simulink model "FOC_CHBI"  (R2025a)
settings: Solver=VariableStepAuto  StartTime=0.0  StopTime=6.5  RelTol=1e-3
InitFcn:
  | %% KHOI THONG SO DONG CO
  | U_nom=6000;%6600;           %dien ap dinh muc dong co
  | H=0.96;%0.9387;             %hieu suat dong co
  | Pn=1e6;%1750e3;         %Cong suat dinh muc dong co
  | cosphi=0.85;%0.9297;        %He so cong suat
  | Sn=Pn/cosphi;       %Cong suat toan phan
  | J=27.9;%34.8;                %Moment quan tinh
  | pc=2;%2;               %So cap cuc
  | fn=50;              %Tan so luoi
  | n=1490;%1486;             %Toc do dinh muc 2880
  | Mdm=6153;%(9.55*Pn*H)/n;  %Moment dinh muc
  | In=117;%Pn/(U_nom*H*cosphi*sqrt(3))   ;
  | Isd=sqrt(2)*In*sqrt(1-cosphi);
  | Isq=sqrt(2*In^2-Isd^2);
  | wrn=2*pi*(fn-(pc*n/60));               %Toc do truotdinh muc
  | Tr=Isq/(wrn*Isd) ;                   %Tinh 'Tr'trong cac cong thuc
  | %Xo=(sqrt(1-cosphi^2)-cosphi*Isd/Isq)*(Un*sqrt(2)/(sqrt(3)*In));
  | Xo=(sqrt(1-cosphi^2)-cosphi*Isd/Isq)*(U_nom/(sqrt(3)*In));
  | Xh=sqrt(2/3)*(U_nom/Isd) - Xo;
  | Rs=(wrn*Isd*Xh)/(2*pi*fn*Isq);
  | Rr=Rs;
  | o=Xo/Xh;
  | Ts=Xh/(2*pi*fn*Rs);
  | Tos=o*Ts;
  | Lr=Tr*Rr;
  | Lor=o*Lr;
  | Ls=Ts*Rs;
  | Los=o*Ls;
  | Lm=sqrt((1-o)*Ls*Lr);
  | %tham so dong co 2850e3Kw
  | %Rs=0.05;
  | %Rr = 0.062;
  | %Los = 0.957/(100*pi);
  | %Lor = 2.237/(100*pi);
  | %Lm = 34.826/(100*pi);
  | %Ts = (Lm +Los)/Rs;
  | %Tr = (Lm+Lor)/Rr;
  | %Lr = Lm + Lor;
  | %Ls = Lm + Los;
  | Udc = 1.1*6000/(0.612*12);%6600/(0.612*12);
  | Rt =18*Udc*Udc/1e6; %18*Udc*Udc/2010.6e3;
  | C_f = 5/(6*100*pi*Rt*0.001);
  | %Fan and Pumb Load Coeficient
  | TL0 = (2.0/100)*Mdm; %(2.0/100)*TN;
  | Omega_rated = n/9.55; %nN/9.55; %rad/s
  | LoadGain = (Mdm - TL0)/(Omega_rated*Omega_rated);
  | fs=5000;
  | %% THAM SO CAC BO DIEU KHIEN
  | %---------------- control volocity
  | epxilon = 0.7;
  | wn = 40;
  |      %P_w = (2*epxilon*wn*J)/pc;
  |     %I_w = wn*wn*J/pc;
  |  P_w = 60;%5;%15;%9;%12;%10;%(2*epxilon*wn*J)/pc
  |  I_w = 80;%150;%80;%100;%40;%50;%wn*wn*J/pc
  | %---------------- control current
  |     %P_id = Rs*Tos*fs/5;
  |     % I_id = Rs*Tos*fs/5/Tos;
  |      %P_iq = P_id;
  |      %I_iq = I_id;
  | P_id = 50;%50;%25;%25;%Rs*Tos*1500/5
  |  I_id = 5000;%5000;%9860;%Rs*Tos*1500/5/Tos
  |  P_iq = 50;%50;%P_id;
  |  I_iq = 5000;%I_id;
  | % --------------control torque
  |  I_phi = 10;%37;%Tr/(5*Tos)/Tr
  |  P_phi = 200;%5;%Tr/(5*Tos)
  |      %I_phi = Tr/(5);
  |      %P_phi = Tr*fs/(5);
StopFcn:
  | figure(1);
  | subplot(1,1,1); hold on; grid on;
  | plot(phi_ref.time, phi_ref.signals.values,'r--', 'Linewidth',1.5);
  | plot(phi.time, phi.signals.values,'b', 'Linewidth',1.5);
  | legend('phi*-rd','phi-rd');
  | title('Từ thông');
  | xlabel('Thời gian (s)'); ylabel('Wb');
  | 
  | 
  | figure(2);
  | subplot(2,1,1); hold on; grid on;
  | plot(torque.time, torque.signals.values,'r','Linewidth',1.5);
  | legend('Te');
  | title('Mô-men');
  | xlabel('Thời gian (s)'); ylabel('Nm');
  | 
  | subplot(2,1,2); hold on; grid on;
  | plot(speed_ref.time, speed_ref.signals.values,'r--','Linewidth',1.5);
  | plot(speed.time, speed.signals.values,'b','Linewidth',1.5);
  | legend('Tốc độ đặt','Tốc độ thực');
  | title('Tốc độ');
  | xlabel('Thời gian (s)'); ylabel('RPM');
  | 
  | figure(3)
  | 
  | subplot(2,1,1); hold on; grid on;
  | plot(isd_ref.time, isd_ref.signals.values,'r','Linewidth',1.5);
  | plot(isd.time, isd.signals.values,'b','Linewidth',1.5);
  | legend('isd*','isd');
  | title('Dòng điện isd');
  | xlabel('Thời gian (s)'); ylabel('A');
  | 
  | subplot(2,1,2); hold on; grid on;
  | plot(isq_ref.time, isq_ref.signals.values,'r','Linewidth',1.5);
  | plot(isq.time, isq.signals.values,'b','Linewidth',1.5);
  | legend('isq*','isq');
  | title('Dòng điện isq');
  | xlabel('Thời gian (s)'); ylabel('A');
  | 
  | figure(4)
  | 
  | subplot(2,1,1); hold on; grid on;
  | plot(va.time, va.signals.values,'b','Linewidth',1.5);
  | plot(vb.time, vb.signals.values,'k','Linewidth',1.5);
  | plot(vc.time, vc.signals.values,'r','Linewidth',1.5);
  | legend('Ua','Ub','Uc');
  | title('Điện áp pha');
  | xlabel('Thời gian (s)'); ylabel('V');
  | 
  | subplot(2,1,2); hold on; grid on;
  | plot(vab.time, vab.signals.values,'k','Linewidth',1.5);
  | plot(vbc.time, vbc.signals.values,'b','Linewidth',1.5);
  | plot(vca.time, vca.signals.values,'r','Linewidth',1.5);
  | legend('Uab','Ubc','Uca');
  | title('Điện áp dây');
  | xlabel('Thời gian (s)'); ylabel('V');
  | 
  | figure(5);
  | subplot(1,1,1); hold on; grid on;
  | plot(Ia.time, Ia.signals.values,'k','Linewidth',1.5);
  | plot(Ib.time, Ib.signals.values,'b','Linewidth',1.5);
  | plot(Ic.time, Ic.signals.values,'r','Linewidth',1.5);
  | legend('Ia','Ib','Ic');
  | title('Dòng điện ba pha của động cơ');
  | xlabel('Thời gian (s)'); ylabel('A');
undefined symbols (not defined in the file): sigbuilder_block
libraries: spsIGBTDiodeLib x72, spsTriangleGeneratorLib x36, spsSeriesRLCBranchLib x18, spsBreakerLib x18, spsUniversalBridgeLib x18, spsZigzagPhaseShiftingTransformerLib x15, spsVoltageMeasurementLib x8, spsACVoltageSourceLib x3, spsCurrentMeasurementLib x3, spsThreePhaseTransformerTwoWindingsLib x3, slpidlib x2, spsThreePhaseVIMeasurementLib x1
(part 1 of 3)
settings Model: Creator=Admin  LastModifiedBy=HP
settings SolverCC: AlgebraicLoopSolver=TrustRegion
settings DataIOCC: ReturnWorkspaceOutputs=off
settings OptimizationCC: ReuseModelBlockBuffer=off
settings DebuggingCC: ArithmeticOperatorsInVariantConditions=warning
settings SFSimCC: CustomCodeUndefinedFunction=UseInterfaceOnly
settings RTWCC: GPUComputeCapability=3.5

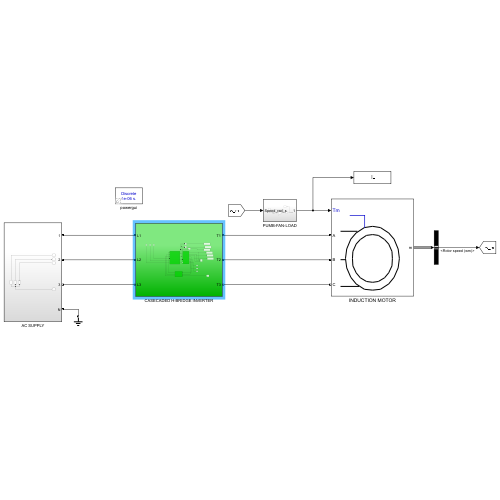
[thumbnail: Simulink's stored preview of the top-level diagram]
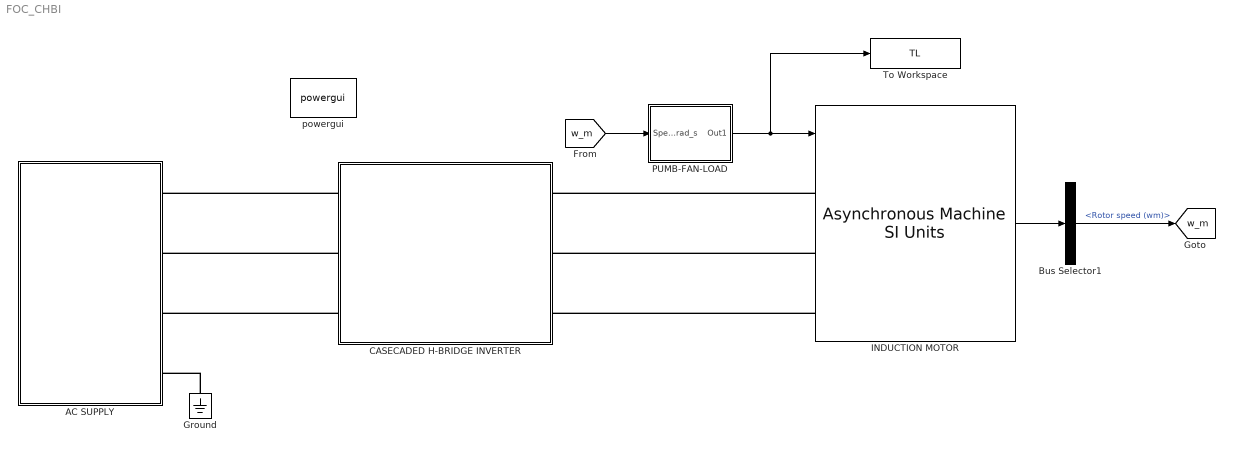
== system FOC_CHBI ==
  AC SUPPLY : Subsystem
  Bus Selector1 : BusSelector  OutputSignals=Mechanical.Rotor speed (wm)
  CASECADED H-BRIDGE INVERTER : Subsystem
  Ground : spsGroundLib/Ground  LConnTagsString=a
  INDUCTION MOTOR : spsAsynchronousMachineSIUnitsLib/Asynchronous Machine SI Units  RotorType=Squirrel-cage  PresetModel=No  MechanicalLoad=Torque Tm  ShowDetailedParameters=on  ReferenceFrame=Rotor  Units=SI  MeasurementBus=off  NominalParameters=[Pn U_nom fn]  VoltageRatio=1  Stator=[Rs Los]  Rotor=[Rr Lor]  Cage1=[ 0.022 0.226/377]  Cage2=[ 0.022 0.226/377]  Lm=Lm  Mechanical=[J 0 pc]  PolePairs=2  InitialConditions=[1,0,0,0,0,0,0,0]  SimulateSaturation=off  Saturation=[0 0;0 0]  LoadFlowParameters=0  TsPowergui=0  TsBlock=-1  IterativeModel=Forward Euler  IterativeDiscreteModel=Trapezoidal non iterative  Pmec=0
      settings: AttributesFormatString=\n
  PUMB-FAN-LOAD : Subsystem
  To Workspace : ToWorkspace  VariableName=TL  SaveFormat=Structure With Time  SampleTime=-1
  powergui : sps_lib/powergui  Priority=1  SimulationMode=Discrete  SampleTime=1e-6  frequency=60  Iterations=50  frequencyindice=0  Pbase=100e6  ErrMax=1e-4  UnitsV=kV  UnitsW=MW  buscounter=0  FunctionMessages=off  echomessages=off  EnableUseOfTLC=off  CurrentSourceSwitches=off  DisableSnubberDevices=off  DisableRonSwitches=off  DisableVfSwitches=off  DisplayEquations=off  AutomaticDiscreteSolvers=off  SolverType=Tustin  Interpol=off  ExternalGateDelay=off  methode=off  Ts=0  x0status=blocks  SPID=on  SwTol=0  HookPort=off  NonlinearTolerance=1e-4  nMaxIteration=100  ContinueOnMaxIteration=off  RestoreLinks=warning  ResistiveCurrentMeasurement=off  Frange=[0:2:500]  Ylog=off  Xlog=on  ShowGrid=off  save=off  variable=ZData  structure=Is  ZoomFFT=off  StartTime=0.8  cycles=5  DisplayStyle=1  fundamental=50  FreqAxis=off  MaxFrequency=1000  frequencyindicesteady=1  RmsSteady=1  display=off
  tag scope: w_m=global
  wires:
  [w_m] -> PUMB-FAN-LOAD/1(Speed_rad_s)
  PUMB-FAN-LOAD/1(Out1) -> To Workspace/1, INDUCTION MOTOR/1
  Bus Selector1/1 -> [w_m]  "<Rotor speed (wm)>"
  INDUCTION MOTOR/1 -> Bus Selector1/1
  connections:
  CASECADED H-BRIDGE INVERTER/LConn3 -- AC SUPPLY/RConn3
  CASECADED H-BRIDGE INVERTER/LConn1 -- AC SUPPLY/RConn1
  INDUCTION MOTOR/LConn2 -- CASECADED H-BRIDGE INVERTER/RConn2
  INDUCTION MOTOR/LConn3 -- CASECADED H-BRIDGE INVERTER/RConn3
  INDUCTION MOTOR/LConn1 -- CASECADED H-BRIDGE INVERTER/RConn1
  Ground/LConn1 -- AC SUPPLY/RConn4
  CASECADED H-BRIDGE INVERTER/LConn2 -- AC SUPPLY/RConn2

== system FOC_CHBI/AC SUPPLY ==
  Va : spsACVoltageSourceLib/AC Voltage Source  Description=source block  Amplitude=sqrt(2)*U_nom/sqrt(3)  Phase=0  Frequency=50  SampleTime=1e-5  Measurements=None  BusType=swing  Pref=10e3  Qref=0  Qmin=-inf  Qmax=+inf
      settings: AttributesFormatString=\n
  Vb : spsACVoltageSourceLib/AC Voltage Source  Description=source block  Amplitude=sqrt(2)*U_nom/sqrt(3)  Phase=-120  Frequency=50  SampleTime=1e-5  Measurements=None  BusType=swing  Pref=10e3  Qref=0  Qmin=-inf  Qmax=+inf
      settings: AttributesFormatString=\n
  Vc : spsACVoltageSourceLib/AC Voltage Source  Description=source block  Amplitude=sqrt(2)*U_nom/sqrt(3)  Phase=120  Frequency=50  SampleTime=1e-5  Measurements=None  BusType=swing  Pref=10e3  Qref=0  Qmin=-inf  Qmax=+inf
      settings: AttributesFormatString=\n
  Connection Port : PMIOPort  Tag=PMCPort  Side=Right
  Connection Port1 : PMIOPort  Tag=PMCPort  Port=2  Side=Right
  Connection Port2 : PMIOPort  Tag=PMCPort  Port=3  Side=Right
  N : PMIOPort  Tag=PMCPort  Port=4  Side=Right
  connections:
  Va/RConn1 -- Connection Port/RConn1
  Vb/RConn1 -- Connection Port1/RConn1
  Vc/RConn1 -- Connection Port2/RConn1
  Va/LConn1 -- N/RConn1 -- Vc/LConn1 -- Vb/LConn1

== system FOC_CHBI/CASECADED H-BRIDGE INVERTER ==
  CONTROLLER : Subsystem
  MEASUREMENT : Subsystem
  POWER CIRCUIT1 : Subsystem
  Scope : Scope  NumInputPorts=3
      settings: Title=Điện áp pha  ActiveDisplayYMinimum=-4924.2153222862125  ActiveDisplayYMaximum=5141.53101611316  YLabel=V
  To Workspace : ToWorkspace  VariableName=vab  SaveFormat=Structure With Time  SampleTime=-1
  To Workspace1 : ToWorkspace  VariableName=va  SaveFormat=Structure With Time  SampleTime=-1
  To Workspace2 : ToWorkspace  VariableName=vbc  SaveFormat=Structure With Time  SampleTime=-1
  To Workspace3 : ToWorkspace  VariableName=vca  SaveFormat=Structure With Time  SampleTime=-1
  To Workspace4 : ToWorkspace  VariableName=vb  SaveFormat=Structure With Time  SampleTime=-1
  To Workspace5 : ToWorkspace  VariableName=vc  SaveFormat=Structure With Time  SampleTime=-1
  Vab : spsVoltageMeasurementLib/Voltage Measurement  PhasorSimulation=off  OutputType=Complex  PSBequivalent=0
  Vbc : spsVoltageMeasurementLib/Voltage Measurement  PhasorSimulation=off  OutputType=Complex  PSBequivalent=0
  Vca : spsVoltageMeasurementLib/Voltage Measurement  PhasorSimulation=off  OutputType=Complex  PSBequivalent=0
  L1 : PMIOPort  Side=Left
  L2 : PMIOPort  Port=2  Side=Left
  L3 : PMIOPort  Port=3  Side=Left
  T1 : PMIOPort  Port=4  Side=Right
  T2 : PMIOPort  Port=5  Side=Right
  T3 : PMIOPort  Port=6  Side=Right
  wires:
  MEASUREMENT/5(iB) -> CONTROLLER/2(Ib)
  [w_m] -> CONTROLLER/3(w)
  MEASUREMENT/4(iA) -> CONTROLLER/1(Ia)
  CONTROLLER/1(phaa) -> POWER CIRCUIT1/1(phaa)
  CONTROLLER/2(phab) -> POWER CIRCUIT1/2(phab)
  CONTROLLER/3(phac) -> POWER CIRCUIT1/3(phac)
  MEASUREMENT/1(Van) -> To Workspace1/1, Scope/1
  MEASUREMENT/2(Vbn) -> Scope/2, To Workspace4/1
  MEASUREMENT/3(Vcn) -> To Workspace5/1, Scope/3
  Vab/1 -> To Workspace/1
  Vbc/1 -> To Workspace2/1
  Vca/1 -> To Workspace3/1
  connections:
  POWER CIRCUIT1/LConn1 -- L1/RConn1
  POWER CIRCUIT1/LConn2 -- L2/RConn1
  POWER CIRCUIT1/LConn3 -- L3/RConn1
  T2/RConn1 -- MEASUREMENT/RConn2
  T3/RConn1 -- MEASUREMENT/RConn3
  T1/RConn1 -- MEASUREMENT/RConn1
  POWER CIRCUIT1/RConn1 -- Vab/LConn1 -- Vca/LConn2 -- MEASUREMENT/LConn1
  POWER CIRCUIT1/RConn2 -- Vab/LConn2 -- Vbc/LConn1 -- MEASUREMENT/LConn2
  POWER CIRCUIT1/RConn3 -- Vbc/LConn2 -- Vca/LConn1 -- MEASUREMENT/LConn3
  POWER CIRCUIT1/RConn4 -- MEASUREMENT/LConn4

== system FOC_CHBI/PUMB-FAN-LOAD ==
  Speed_rad_s : Inport
  Add : Sum
  Constant1 : Constant  Value=TL0
  Gain : Gain  Gain=LoadGain
  Product : Product
  Out1 : Outport  VectorParamsAs1DForOutWhenUnconnected=off
  tag scope: TL=global
  wires:
  Constant1/1 -> Add/1
  Product/1 -> Gain/1
  Gain/1 -> Add/2
  Add/1 -> [TL], Out1/1
  Speed_rad_s/1 -> Product/1, Product/2

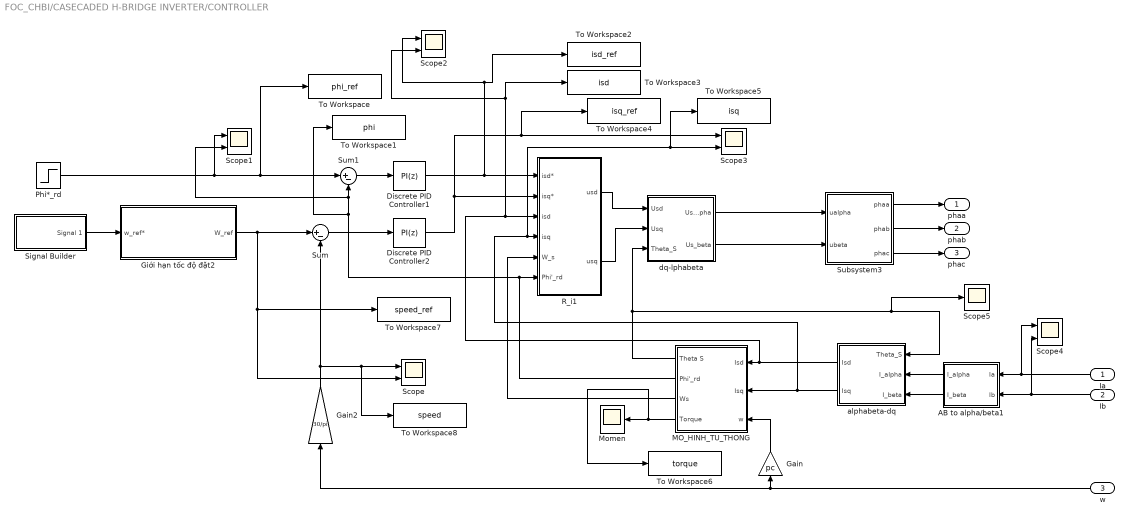
== system FOC_CHBI/CASECADED H-BRIDGE INVERTER/CONTROLLER ==
  Ia : Inport
  Ib : Inport  Port=2
  w : Inport  Port=3
  AB to alpha/beta1 : Subsystem
  Discrete PID Controller1 : slpidlib/PID Controller  Controller=PI  Form=Parallel  TimeDomain=Discrete-time  UseExternalTs=off  SampleTime=1/5e5  IntegratorMethod=Forward Euler  FilterMethod=Forward Euler  ControllerParametersSource=internal  P=P_phi  I=I_phi  UseKiTs=off  D=0  UseExternalDerivativeSource=off  N=100  UseFilter=on  TunerSelectOption=Transfer Function Based (PID Tuner App)  InitialConditionSource=internal  InitialConditionForIntegrator=0  InitialConditionForFilter=0  DifferentiatorICPrevScaledInput=0  ExternalReset=none  TrackingMode=off  Kt=1  LimitOutput=on  SatLimitsSource=internal  UpperSaturationLimit=1.8*Isd  LowerSaturationLimit=-1.8*Isd  LinearizeAsGain=off  AntiWindupMode=clamping  Kb=1  LimitIntegrator=off  UpperIntegratorSaturationLimit=inf  LowerIntegratorSaturationLimit=-inf  POutMin=[]  POutMax=[]  IOutMin=[]  IOutMax=[]  DOutMin=[]  DOutMax=[]  NOutMin=[]  NOutMax=[]  SumOutMin=[]  SumOutMax=[]  SaturationOutMin=[]  SaturationOutMax=[]  PParamMin=[]  PParamMax=[]  IParamMin=[]  IParamMax=[]  DParamMin=[]  DParamMax=[]  NParamMin=[]  NParamMax=[]  KbParamMin=[]  KbParamMax=[]  KtParamMin=[]  KtParamMax=[]  KbOutMin=[]  KbOutMax=[]  KtOutMin=[]  KtOutMax=[]  IntegratorOutMin=[]  IntegratorOutMax=[]  FilterOutMin=[]  FilterOutMax=[]  SumI1OutMin=[]  SumI1OutMax=[]  SumI2OutMin=[]  SumI2OutMax=[]  SumI3OutMin=[]  SumI3OutMax=[]  SumI4OutMin=[]  SumI4OutMax=[]  SumDOutMin=[]  SumDOutMax=[]  DifferentiatorOutMin=[]  DifferentiatorOutMax=[]  FilterDiffOutCoefMin=[]  FilterDiffOutCoefMax=[]  ReciprocalOutMin=[]  ReciprocalOutMax=[]  SumDenOutMin=[]  SumDenOutMax=[]  SumNumOutMin=[]  SumNumOutMax=[]  DivideOutMin=[]  DivideOutMax=[]  UdiffTsProdOutMin=[]  UdiffTsProdOutMax=[]  NTsProdOutMin=[]  NTsProdOutMax=[]  UintegralTsProdOutMin=[]  UintegralTsProdOutMax=[]  UngainTsProdOutMin=[]  UngainTsProdOutMax=[]  ClampingZeroOutDataTypeStr=Inherit: Inherit via back propagation  ClampingZeroOutMin=[]  ClampingZeroOutMax=[]  FilterDenConstantOutDataTypeStr=Inherit: Inherit via back propagation  FilterDenConstantOutMin=[]  FilterDenConstantOutMax=[]  PCopyOutDataTypeStr=Inherit: Inherit via back propagation  PCopyOutMin=[]  PCopyOutMax=[]  NCopyOutDataTypeStr=Inherit: Inherit via back propagation  NCopyOutMin=[]  NCopyOutMax=[]  IntegratorContinuousStateAttributes=''  IntegratorStateMustResolveToSignalObject=off  IntegratorRTWStateStorageClass=Auto  FilterContinuousStateAttributes=''  FilterStateMustResolveToSignalObject=off  FilterRTWStateStorageClass=Auto  ParallelPVariant=InternalParameters  IdealPVariant=Disabled  IVariant=InternalParameters  DVariant=Disabled  IntegratorVariant=Discrete  SatVariant=Enabled  AWVariant=DiscClampingParallel  PCopyVariant=Disabled  TRVariant=Disabled  FdbkBlocksVariant=Forward  IdealPFdbkVariant=Disabled  SatFdbkVariant=Disabled  DerivativeFilterVariant=Disabled  NVariant=Disabled  NCopyVariant=Disabled_SignalSpec  FilterICVariant=Disabled  IntegratorICVariant=InternalICs  ExternalResetVariant=Disabled  TRSumVariant=Passthrough  SumFdbkVariant=Disabled  SumVariant=Sum_PI  TsampFilterVariant=InternalTs  TsampNgainVariant=Passthrough  TsampIntegralVariant=Disabled_SignalSpec  ExternalSaturationOutDataTypeStr=Inherit: Same as second input  DerivativeSourceVariant=Disabled  PreIntVariant=InternalPreInt
  Discrete PID Controller2 : slpidlib/PID Controller  Controller=PI  Form=Parallel  TimeDomain=Discrete-time  UseExternalTs=off  SampleTime=1/5e5  IntegratorMethod=Forward Euler  FilterMethod=Forward Euler  ControllerParametersSource=internal  P=P_w  I=I_w  UseKiTs=off  D=0  UseExternalDerivativeSource=off  N=100  UseFilter=on  TunerSelectOption=Transfer Function Based (PID Tuner App)  InitialConditionSource=internal  InitialConditionForIntegrator=0  InitialConditionForFilter=0  DifferentiatorICPrevScaledInput=0  ExternalReset=none  TrackingMode=off  Kt=1  LimitOutput=on  SatLimitsSource=internal  UpperSaturationLimit=1.5*Isq  LowerSaturationLimit=-1.5*Isq  LinearizeAsGain=off  AntiWindupMode=none  Kb=1  LimitIntegrator=off  UpperIntegratorSaturationLimit=inf  LowerIntegratorSaturationLimit=-inf  POutMin=[]  POutMax=[]  IOutMin=[]  IOutMax=[]  DOutMin=[]  DOutMax=[]  NOutMin=[]  NOutMax=[]  SumOutMin=[]  SumOutMax=[]  SaturationOutMin=[]  SaturationOutMax=[]  PParamMin=[]  PParamMax=[]  IParamMin=[]  IParamMax=[]  DParamMin=[]  DParamMax=[]  NParamMin=[]  NParamMax=[]  KbParamMin=[]  KbParamMax=[]  KtParamMin=[]  KtParamMax=[]  KbOutMin=[]  KbOutMax=[]  KtOutMin=[]  KtOutMax=[]  IntegratorOutMin=[]  IntegratorOutMax=[]  FilterOutMin=[]  FilterOutMax=[]  SumI1OutMin=[]  SumI1OutMax=[]  SumI2OutMin=[]  SumI2OutMax=[]  SumI3OutMin=[]  SumI3OutMax=[]  SumI4OutMin=[]  SumI4OutMax=[]  SumDOutMin=[]  SumDOutMax=[]  DifferentiatorOutMin=[]  DifferentiatorOutMax=[]  FilterDiffOutCoefMin=[]  FilterDiffOutCoefMax=[]  ReciprocalOutMin=[]  ReciprocalOutMax=[]  SumDenOutMin=[]  SumDenOutMax=[]  SumNumOutMin=[]  SumNumOutMax=[]  DivideOutMin=[]  DivideOutMax=[]  UdiffTsProdOutMin=[]  UdiffTsProdOutMax=[]  NTsProdOutMin=[]  NTsProdOutMax=[]  UintegralTsProdOutMin=[]  UintegralTsProdOutMax=[]  UngainTsProdOutMin=[]  UngainTsProdOutMax=[]  ClampingZeroOutDataTypeStr=Inherit: Inherit via back propagation  ClampingZeroOutMin=[]  ClampingZeroOutMax=[]  FilterDenConstantOutDataTypeStr=Inherit: Inherit via back propagation  FilterDenConstantOutMin=[]  FilterDenConstantOutMax=[]  PCopyOutDataTypeStr=Inherit: Inherit via back propagation  PCopyOutMin=[]  PCopyOutMax=[]  NCopyOutDataTypeStr=Inherit: Inherit via back propagation  NCopyOutMin=[]  NCopyOutMax=[]  IntegratorContinuousStateAttributes=''  IntegratorStateMustResolveToSignalObject=off  IntegratorRTWStateStorageClass=Auto  FilterContinuousStateAttributes=''  FilterStateMustResolveToSignalObject=off  FilterRTWStateStorageClass=Auto  ParallelPVariant=InternalParameters  IdealPVariant=Disabled  IVariant=InternalParameters  DVariant=Disabled  IntegratorVariant=Discrete  SatVariant=Enabled  AWVariant=Passthrough  PCopyVariant=Disabled  TRVariant=Disabled  FdbkBlocksVariant=Forward  IdealPFdbkVariant=Disabled  SatFdbkVariant=Disabled  DerivativeFilterVariant=Disabled  NVariant=Disabled  NCopyVariant=Disabled_SignalSpec  FilterICVariant=Disabled  IntegratorICVariant=InternalICs  ExternalResetVariant=Disabled  TRSumVariant=Passthrough  SumFdbkVariant=Disabled  SumVariant=Sum_PI  TsampFilterVariant=InternalTs  TsampNgainVariant=Passthrough  TsampIntegralVariant=Disabled_SignalSpec  ExternalSaturationOutDataTypeStr=Inherit: Same as second input  DerivativeSourceVariant=Disabled  PreIntVariant=InternalPreInt
  Gain : Gain  Gain=pc
  Gain2 : Gain  Gain=30/pi
  Giới hạn tốc độ đặt2 : Subsystem
  MO_HINH_TU_THONG : Subsystem
  Momen : Scope
      settings: TimeSpan=1  Title=Mô men  ActiveDisplayYMinimum=-3672.60533  ActiveDisplayYMaximum=33053.44795  YLabel=Nm  DataLoggingVariableName=m1
  Phi*_rd : Step  Time=0  Before=0.0001  After=Isd  SampleTime=1e-5  ZeroCross=off
  R_i1 : Subsystem
  Scope{,1..4} (5 alike) : Scope  NumInputPorts=2
      Scope settings: Title=Tốc độ động cơ  ActiveDisplayYMinimum=-128.51639  ActiveDisplayYMaximum=1116.50182  YLabel=Vòng/phút  DataLoggingVariableName=ScopeData4
      Scope1 settings: Title=Từ thông  ActiveDisplayYMinimum=-23.37354  ActiveDisplayYMaximum=210.3619  YLabel=wb  DataLoggingVariableName=ScopeData5
      Scope2 settings: Title=Dòng điện Isd  ActiveDisplayYMinimum=63.502062069951819  ActiveDisplayYMaximum=63.993054341937629  YLabel=A
      Scope3 settings: Title=Dòng điện Isq  ActiveDisplayYMinimum=71.311410878345953  ActiveDisplayYMaximum=72.655332560271432  YLabel=A  DataLoggingVariableName=ScopeData2
      Scope4 settings: ActiveDisplayYMinimum=-637.9246  ActiveDisplayYMaximum=637.49207
  Scope5 : Scope
      settings: ActiveDisplayYMinimum=-132.92462  ActiveDisplayYMaximum=1196.32155  DataLoggingVariableName=ScopeData2
  Signal Builder : Subsystem  Tag=STV Subsys  LoadFcn=sigbuilder_block('load');  StartFcn=sigbuilder_block('start');  StopFcn=sigbuilder_block('stop');  ClipboardFcn=sigbuilder_block('clipboard');  mask(Sigbuilder block){tuvar=[0:10]}
      mask help: Simulink:masks:SigbuilderBlock_MD
      mask init:
      | if ~strcmp(get_param(bdroot(gcbh),'SimulationStatus'),'stopped') tuvar = sigbuilder_block('maskInit'); end
      settings: CopyFcn=sigbuilder_block('copy');  DeleteFcn=sigbuilder_block('delete');  ModelCloseFcn=sigbuilder_block('modelClose');  PreSaveFcn=sigbuilder_block('preSave');  PauseFcn=sigbuilder_block('pause');  ContinueFcn=sigbuilder_block('continue');  NameChangeFcn=sigbuilder_block('namechange');  OpenFcn=sigbuilder_block('open',[316.5 171.75 805.5 485.25 ]);  CloseFcn=sigbuilder_block('close');
      mask Display: plot(0, 0, 100, 100,[2, 2, 32, 32, 2], [68, 8, 8, 68, 68],[32, 2], [38, 38], [32, 19, 2],[53, 60, 44], [32, 17, 17, 2],[16, 16, 31, 31]);txt = getActiveGroup(gcbh);text(2, 100, txt,'verticalAlignment', 'top');
  Subsystem3 : Subsystem
  Sum : Sum  Inputs=|+-
  Sum1 : Sum  Inputs=|+-
  To Workspace : ToWorkspace  VariableName=phi_ref  SaveFormat=Structure With Time  SampleTime=-1
  To Workspace1 : ToWorkspace  VariableName=phi  SaveFormat=Structure With Time  SampleTime=-1
  To Workspace2 : ToWorkspace  VariableName=isd_ref  SaveFormat=Structure With Time  SampleTime=-1
  To Workspace3 : ToWorkspace  VariableName=isd  SaveFormat=Structure With Time  SampleTime=-1
  To Workspace4 : ToWorkspace  VariableName=isq_ref  SaveFormat=Structure With Time  SampleTime=-1
  To Workspace5 : ToWorkspace  VariableName=isq  SaveFormat=Structure With Time  SampleTime=-1
  To Workspace6 : ToWorkspace  VariableName=torque  SaveFormat=Structure With Time  SampleTime=-1
  To Workspace7 : ToWorkspace  VariableName=speed_ref  SaveFormat=Structure With Time  SampleTime=-1
  To Workspace8 : ToWorkspace  VariableName=speed  SaveFormat=Structure With Time  SampleTime=-1
  "alphabeta-dq  " : Subsystem
  dq-lphabeta : Subsystem
  phaa : Outport
  phab : Outport  Port=2
  phac : Outport  Port=3
  wires:
  R_i1/2(usq) -> dq-lphabeta/2(Usq)
  MO_HINH_TU_THONG/4("Torque ") -> To Workspace6/1, Momen/1
  dq-lphabeta/2("Us_beta ") -> Subsystem3/2(ubeta)
  Gain/1 -> MO_HINH_TU_THONG/3(w)
  dq-lphabeta/1(Us_alpha) -> Subsystem3/1(ualpha)
  "alphabeta-dq  "/2(Isq) -> MO_HINH_TU_THONG/2(Isq), To Workspace5/1, Scope3/2, R_i1/4(isq)
  MO_HINH_TU_THONG/1(Theta S) -> dq-lphabeta/3(Theta_S), Scope5/1, "alphabeta-dq  "/1(Theta_S)
  MO_HINH_TU_THONG/2(Phi'_rd) -> To Workspace1/1, Scope1/2, Sum1/2, R_i1/6(Phi'_rd)
  w/1 -> Gain/1, Gain2/1
  MO_HINH_TU_THONG/3(Ws) -> R_i1/5(W_s)
  R_i1/1(usd) -> dq-lphabeta/1(Usd)
  Phi*_rd/1 -> Scope1/1, To Workspace/1, Sum1/1
  Gain2/1 -> Sum/2, To Workspace8/1, Scope/1
  AB to alpha/beta1/2(I_beta) -> "alphabeta-dq  "/3(I_beta)
  AB to alpha/beta1/1(I_alpha) -> "alphabeta-dq  "/2(I_alpha)
  Ib/1 -> Scope4/2, AB to alpha/beta1/2(Ib)
  Subsystem3/1(phaa) -> phaa/1
  Subsystem3/2(phab) -> phab/1
  Subsystem3/3(phac) -> phac/1
  Signal Builder/1(Signal 1) -> Giới hạn tốc độ đặt2/1(w_ref*)
  Giới hạn tốc độ đặt2/1(W_ref) -> To Workspace7/1, Scope/2, Sum/1
  Ia/1 -> Scope4/1, AB to alpha/beta1/1(Ia)
  Sum1/1 -> Discrete PID Controller1/1
  Sum/1 -> Discrete PID Controller2/1
  Discrete PID Controller1/1 -> To Workspace2/1, Scope2/1, R_i1/1(isd*)
  Discrete PID Controller2/1 -> To Workspace4/1, Scope3/1, R_i1/2(isq*)
  "alphabeta-dq  "/1(Isd) -> MO_HINH_TU_THONG/1(Isd), R_i1/3(isd), To Workspace3/1, Scope2/2

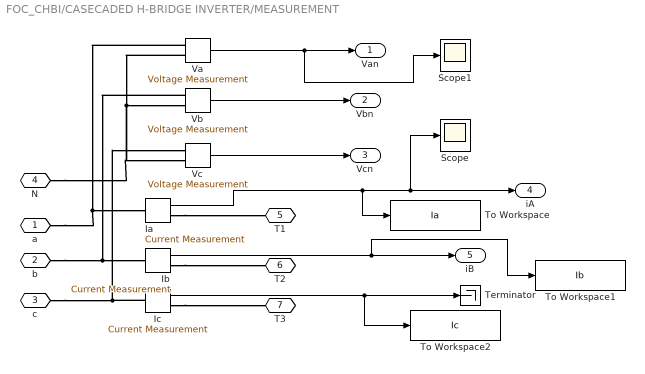
== system FOC_CHBI/CASECADED H-BRIDGE INVERTER/MEASUREMENT ==
  Ia : spsCurrentMeasurementLib/Current Measurement  PhasorSimulation=off  OutputType=Complex  PSBequivalent=0
  Ib : spsCurrentMeasurementLib/Current Measurement  PhasorSimulation=off  OutputType=Complex  PSBequivalent=0
  Ic : spsCurrentMeasurementLib/Current Measurement  PhasorSimulation=off  OutputType=Complex  PSBequivalent=0
  Scope : Scope
      settings: ActiveDisplayYMinimum=-651.81083  ActiveDisplayYMaximum=651.79585  DataLoggingVariableName=ia
  Scope1 : Scope
      settings: ActiveDisplayYMinimum=-6719.10332  ActiveDisplayYMaximum=6719.01889  DataLoggingVariableName=Van
  Terminator : Terminator
  To Workspace : ToWorkspace  VariableName=Ia  SaveFormat=Structure With Time  SampleTime=-1
  To Workspace1 : ToWorkspace  VariableName=Ib  SaveFormat=Structure With Time  SampleTime=-1
  To Workspace2 : ToWorkspace  VariableName=Ic  SaveFormat=Structure With Time  SampleTime=-1
  Va : spsVoltageMeasurementLib/Voltage Measurement  PhasorSimulation=off  OutputType=Complex  PSBequivalent=0
  Vb : spsVoltageMeasurementLib/Voltage Measurement  PhasorSimulation=off  OutputType=Complex  PSBequivalent=0
  Vc : spsVoltageMeasurementLib/Voltage Measurement  PhasorSimulation=off  OutputType=Complex  PSBequivalent=0
  a : PMIOPort  Side=Left
  b : PMIOPort  Port=2  Side=Left
  c : PMIOPort  Port=3  Side=Left
  N : PMIOPort  Port=4  Side=Left
  T1 : PMIOPort  Port=5  Side=Right
  T2 : PMIOPort  Port=6  Side=Right
  T3 : PMIOPort  Port=7  Side=Right
  Van : Outport
  Vbn : Outport  Port=2
  Vcn : Outport  Port=3
  iA : Outport  Port=4
  iB : Outport  Port=5
  wires:
  Ic/1 -> To Workspace2/1, Terminator/1
  Va/1 -> Scope1/1, Van/1
  Ib/1 -> To Workspace1/1, iB/1
  Ia/1 -> To Workspace/1, Scope/1, iA/1
  Vb/1 -> Vbn/1
  Vc/1 -> Vcn/1
  connections:
  Ic/LConn1 -- Vc/LConn1 -- c/RConn1
  Va/LConn2 -- N/RConn1 -- Vc/LConn2 -- Vb/LConn2
  Ia/RConn1 -- T1/RConn1
  Ib/RConn1 -- T2/RConn1
  Va/LConn1 -- Ia/LConn1 -- a/RConn1
  Vb/LConn1 -- Ib/LConn1 -- b/RConn1
  Ic/RConn1 -- T3/RConn1

== system FOC_CHBI/CASECADED H-BRIDGE INVERTER/POWER CIRCUIT1 ==
  phaa : Inport
  phab : Inport  Port=2
  phac : Inport  Port=3
  Gate state1 : Subsystem
  "Gate state2 " : Subsystem
  Gate state3 : Subsystem
  Subsystem : Subsystem
  Subsystem1 : Subsystem
  Subsystem2 : Subsystem
  A : PMIOPort  Side=Left
  B : PMIOPort  Port=2  Side=Left
  C : PMIOPort  Port=3  Side=Left
  "a " : PMIOPort  Port=4  Side=Right
  b : PMIOPort  Port=5  Side=Right
  c : PMIOPort  Port=6  Side=Right
  N : PMIOPort  Port=7  Side=Right
  wires:
  phac/1 -> Gate state3/1(phac)
  phab/1 -> "Gate state2 "/1(phab)
  phaa/1 -> Gate state1/1(phaa)
  Gate state3/4(GateH4) -> Subsystem1/4(Inport3)
  Gate state1/6(GateH6) -> Subsystem2/6(Inport5)
  Gate state3/1(GateH1) -> Subsystem1/1(Inport)
  Gate state3/5(GateH5) -> Subsystem1/5(Inport4)
  "Gate state2 "/5(GateH5) -> Subsystem/5(Inport4)
  "Gate state2 "/4(GateH4) -> Subsystem/4(Inport3)
  Gate state3/2(GateH2) -> Subsystem1/2(Inport1)
  "Gate state2 "/2(GateH2) -> Subsystem/2(Inport1)
  Gate state3/3(GateH3) -> Subsystem1/3(Inport2)
  "Gate state2 "/3(GateH3) -> Subsystem/3(Inport2)
  Gate state1/1(GateH1) -> Subsystem2/1(Inport)
  Gate state1/3(GateH3) -> Subsystem2/3(Inport2)
  "Gate state2 "/1(GateH1) -> Subsystem/1(Inport)
  Gate state1/5(GateH5) -> Subsystem2/5(Inport4)
  Gate state3/6(GateH6) -> Subsystem1/6(Inport5)
  Gate state1/4(GateH4) -> Subsystem2/4(Inport3)
  Gate state1/2(GateH2) -> Subsystem2/2(Inport1)
  "Gate state2 "/6(GateH6) -> Subsystem/6(Inport5)
  connections:
  N/RConn1 -- Subsystem1/LConn2 -- Subsystem2/LConn2 -- Subsystem/LConn2
  c/RConn1 -- Subsystem1/LConn1
  b/RConn1 -- Subsystem/LConn1
  Subsystem2/LConn1 -- "a "/RConn1
  A/RConn1 -- Subsystem2/LConn3 -- Subsystem/LConn3 -- Subsystem1/LConn3
  C/RConn1 -- Subsystem2/LConn5 -- Subsystem/LConn5 -- Subsystem1/LConn5
  B/RConn1 -- Subsystem2/LConn4 -- Subsystem1/LConn4 -- Subsystem/LConn4

== system FOC_CHBI/CASECADED H-BRIDGE INVERTER/CONTROLLER/AB to alpha//beta1 ==
  Ia : Inport
  Ib : Inport  Port=2
  Gain : Gain  Gain=2
  Gain1 : Gain  Gain=1/sqrt(3)
  Sum : Sum  Inputs=++|
  I_alpha : Outport
  I_beta : Outport  Port=2
  wires:
  Ia/1 -> Sum/1, I_alpha/1
  Ib/1 -> Gain/1
  Gain/1 -> Sum/2
  Sum/1 -> Gain1/1
  Gain1/1 -> I_beta/1

== system FOC_CHBI/CASECADED H-BRIDGE INVERTER/CONTROLLER/Giới hạn tốc độ đặt2 ==
  w_ref* : Inport
  1 : Constant  Value=0.95
  Constant1 : Constant
  Constant2 : Constant  Value=4*Udc*sqrt(3)  SampleTime=1e-5
  MATLAB Function1 : MATLAB Function  TreatAsAtomicUnit=on
  Mux : Mux  Inputs=3
  Product : Product
  Scope : Scope
      settings: ActiveDisplayYMinimum=-124  ActiveDisplayYMaximum=1116
  Step : Step  Time=4  Before=1  After=-1  SampleTime=0
  Switch : Switch  Criteria=u2 > Threshold  SaturateOnIntegerOverflow=off  InputSameDT=off
  Transfer Fcn1 : TransferFcn  Denominator=[0.04 1]
  error : Subsystem
  W_ref : Outport
  wires:
  Constant2/1 -> MATLAB Function1/1(Umax)
  w_ref*/1 -> MATLAB Function1/3(v_ref)
  1/1 -> Switch/3
  Product/1 -> Transfer Fcn1/1, Scope/1
  MATLAB Function1/1(vt) -> Product/2
  Switch/1 -> Product/1
  Step/1 -> Switch/2
  Constant1/1 -> Switch/1
  Transfer Fcn1/1 -> W_ref/1
  error/1(errorA) -> Mux/1
  error/2(errorB) -> Mux/2
  error/3(errorC) -> Mux/3
  Mux/1 -> MATLAB Function1/2(e)

== system FOC_CHBI/CASECADED H-BRIDGE INVERTER/CONTROLLER/MO_HINH_TU_THONG ==
  note: Wr
  Isd : Inport
  Isq : Inport  Port=2
  w : Inport  Port=3
  Constant : Constant  Value=1e-6  SampleTime=1e-5
  Divide : Product  Inputs=/*
  Gain1 : Gain  Gain=(3/2)*pc*Lm*Lm/Lr
  Gain2 : Gain  Gain=1/Tr
  Integrator : Integrator
  Product : Product
  Sum : Sum  Inputs=|++
  Sum1 : Sum  Inputs=|++
  Transfer Fcn : TransferFcn  Denominator=[Tr 1]
  Theta S : Outport
  Phi'_rd : Outport  Port=2
  Ws : Outport  Port=3
  "Torque " : Outport  Port=4
  wires:
  Transfer Fcn/1 -> Sum1/1, Product/1, Phi'_rd/1
  Divide/1 -> Sum/1
  w/1 -> Sum/2
  Integrator/1 -> Theta S/1
  Sum/1 -> Integrator/1, Ws/1
  Isd/1 -> Transfer Fcn/1
  Product/1 -> Gain1/1
  Gain1/1 -> "Torque "/1
  Sum1/1 -> Divide/1
  Isq/1 -> Product/2, Gain2/1
  Gain2/1 -> Divide/2
  Constant/1 -> Sum1/2

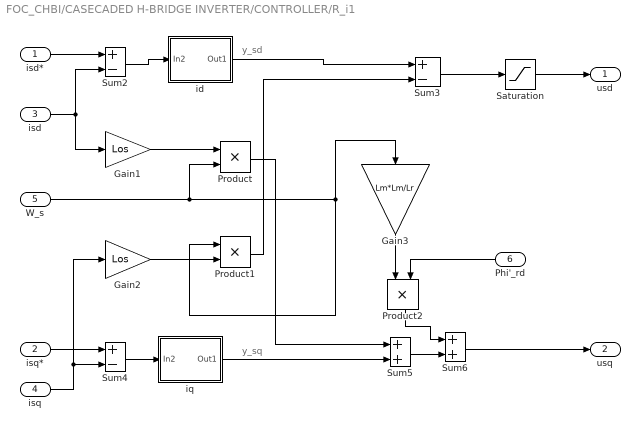
== system FOC_CHBI/CASECADED H-BRIDGE INVERTER/CONTROLLER/R_i1 ==
  note: y_sq
  note: y_sd
  isd* : Inport
  isq* : Inport  Port=2
  isd : Inport  Port=3
  isq : Inport  Port=4
  W_s : Inport  Port=5
  Phi'_rd : Inport  Port=6
  Gain1 : Gain  Gain=Los
  Gain2 : Gain  Gain=Los
  Gain3 : Gain  Gain=Lm*Lm/Lr
  Product : Product  RndMeth=Zero
  Product1 : Product  RndMeth=Zero
  Product2 : Product  RndMeth=Zero
  Saturation : Saturate  UpperLimit=U_nom  LowerLimit=-U_nom
  Sum2 : Sum  Inputs=+-
  Sum3 : Sum  Inputs=+-
  Sum4 : Sum  Inputs=+-
  Sum5 : Sum
  Sum6 : Sum
  id : Subsystem  mask{Kp=P_id*5*10, Ki=10*I_id/20, T=1/5e5, limit=1000}
      mask prompts: T "Sample time"
  iq : Subsystem  mask{Kp=P_iq*5*10, Ki=10*I_iq/20, T=1/5e5, limit=1000}
      mask prompts: T "Sample time"
  usd : Outport  InitialOutput=0
  usq : Outport  Port=2  InitialOutput=0
  wires:
  Sum4/1 -> iq/1(In2)
  isd*/1 -> Sum2/1
  Gain3/1 -> Product2/1
  W_s/1 -> Gain3/1, Product1/1, Product/2
  Product1/1 -> Sum3/2
  Phi'_rd/1 -> Product2/2
  iq/1(Out1) -> Sum5/2
  isq/1 -> Gain2/1, Sum4/2
  Gain1/1 -> Product/1
  Sum3/1 -> Saturation/1
  Product/1 -> Sum5/1
  isd/1 -> Gain1/1, Sum2/2
  isq*/1 -> Sum4/1
  Product2/1 -> Sum6/1
  Sum2/1 -> id/1(In2)
  Gain2/1 -> Product1/2
  Sum6/1 -> usq/1
  Sum5/1 -> Sum6/2
  Saturation/1 -> usd/1
  id/1(Out1) -> Sum3/1

== system FOC_CHBI/CASECADED H-BRIDGE INVERTER/CONTROLLER/Signal Builder ==
  Demux : Demux  Tag=STV Demux  Outputs=1
      settings: DisplayOption=none
  FromWs : FromWorkspace  Tag=STV FromWs  VariableName=tuvar
      SigBuilderData=|
      | common.afterFinalStr = 'Extrapolate'
      | common.sampleTime = 0
      | dataSet.timeRange = [0 7]
      | dataSet.name = 'Group 1'
      | sbobj.Groups.Name = 'Group 1'
      | sbobj.Groups.Signals.Name = 'Signal 1'
      | sbobj.Groups.Signals.XData = [0 0.4 0.8 1.15 2.5 3 3.5 4.5 5 7]
      | sbobj.Groups.Signals.YData = [0 0 0 200 992 992 992 992 992 992]
      | sbobj.Groups.TimeRange = [0 7]
  Signal 1 : Outport  Tag=STV Outport
  wires:
  FromWs/1 -> Demux/1
  Demux/1 -> Signal 1/1

== system FOC_CHBI/CASECADED H-BRIDGE INVERTER/CONTROLLER/Subsystem3 ==
  ualpha : Inport
  ubeta : Inport  Port=2
  Gain : Gain  Gain=1/2
  Gain1 : Gain  Gain=sqrt(3)/2
  Gain2 : Gain  Gain=1/(6*Udc)
  Gain3 : Gain  Gain=1/(6*Udc)
  Gain4 : Gain  Gain=1/(6*Udc)
  Sum : Sum  Inputs=|-+
  Sum1 : Sum  Inputs=|--
  phaa : Outport
  phab : Outport  Port=2
  phac : Outport  Port=3
  wires:
  Gain4/1 -> phac/1
  Gain3/1 -> phab/1
  Sum/1 -> Gain3/1
  Gain2/1 -> phaa/1
  Gain1/1 -> Sum/2, Sum1/2
  Gain/1 -> Sum/1, Sum1/1
  ualpha/1 -> Gain2/1, Gain/1
  Sum1/1 -> Gain4/1
  ubeta/1 -> Gain1/1

== system FOC_CHBI/CASECADED H-BRIDGE INVERTER/CONTROLLER/alphabeta-dq   ==
  Theta_S : Inport
  I_alpha : Inport  Port=2
  I_beta : Inport  Port=3
  Gain1 : Gain  Gain=-1
  Product{,1..3} (4 alike) : Product
  Sum : Sum  Inputs=|++|
  Sum1 : Sum  Inputs=|++|
  Trigonometric Function : Trigonometry
  Trigonometric Function1 : Trigonometry  Operator=cos
  Isd : Outport  InitialOutput=0
  Isq : Outport  Port=2  InitialOutput=0
  wires:
  Trigonometric Function1/1 -> Product/2, Product3/2
  I_beta/1 -> Product3/1, Product1/1
  Trigonometric Function/1 -> Product2/2, Product1/2
  Product/1 -> Sum/1
  Product1/1 -> Sum/2
  Sum/1 -> Isd/1
  I_alpha/1 -> Product/1, Gain1/1
  Gain1/1 -> Product2/1
  Product2/1 -> Sum1/1
  Product3/1 -> Sum1/2
  Sum1/1 -> Isq/1
  Theta_S/1 -> Trigonometric Function1/1, Trigonometric Function/1

== system FOC_CHBI/CASECADED H-BRIDGE INVERTER/CONTROLLER/dq-lphabeta ==
  Usd : Inport
  Usq : Inport  Port=2
  Theta_S : Inport  Port=3
  Product{,1..3} (4 alike) : Product
  Sum : Sum  Inputs=|+-
  Sum1 : Sum  Inputs=|++
  Trigonometric Function : Trigonometry
  Trigonometric Function1 : Trigonometry  Operator=cos
  Us_alpha : Outport  InitialOutput=0
  "Us_beta " : Outport  Port=2  InitialOutput=0
  wires:
  Usd/1 -> Product/2, Product3/1
  Product/1 -> Sum/1
  Product1/1 -> Sum/2
  Usq/1 -> Product2/1, Product1/1
  Sum/1 -> Us_alpha/1
  Product2/1 -> Sum1/1
  Product3/1 -> Sum1/2
  Sum1/1 -> "Us_beta "/1
  Trigonometric Function1/1 -> Product/1, Product2/2
  Trigonometric Function/1 -> Product3/2, Product1/2
  Theta_S/1 -> Trigonometric Function/1, Trigonometric Function1/1

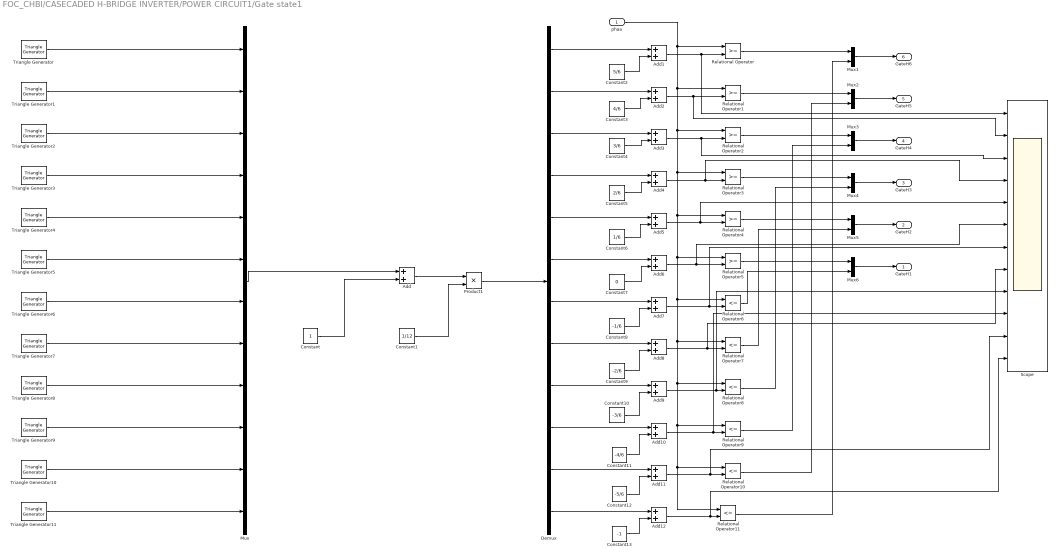
== system FOC_CHBI/CASECADED H-BRIDGE INVERTER/POWER CIRCUIT1/Gate state1 ==
  phaa : Inport
  Add{,1..12} (13 alike) : Sum
  Constant : Constant  SampleTime=1e-5
  Constant1 : Constant  Value=1/12  SampleTime=1e-5
  Constant10 : Constant  Value=-3/6  SampleTime=1e-5
  Constant11 : Constant  Value=-4/6  SampleTime=1e-5
  Constant12 : Constant  Value=-5/6  SampleTime=1e-5
  Constant13 : Constant  Value=-1  SampleTime=1e-5
  Constant2 : Constant  Value=5/6  SampleTime=1e-5
  Constant3 : Constant  Value=4/6  SampleTime=1e-5
  Constant4 : Constant  Value=3/6  SampleTime=1e-5
  Constant5 : Constant  Value=2/6  SampleTime=1e-5
  Constant6 : Constant  Value=1/6  SampleTime=1e-5
  Constant7 : Constant  Value=0  SampleTime=1e-5
  Constant8 : Constant  Value=-1/6  SampleTime=1e-5
  Constant9 : Constant  Value=-2/6  SampleTime=1e-5
  Demux : Demux  Outputs=12
  Mux : Mux  Inputs=12
  Mux{1..6} (6 alike) : Mux  Inputs=2
  Product1 : Product
  Relational Operator{,1..5} (6 alike) : RelationalOperator  OutDataTypeStr=boolean  InputSameDT=off
  Relational Operator{6..11} (6 alike) : RelationalOperator  Operator=<=  OutDataTypeStr=boolean  InputSameDT=off
  Scope : Scope  NumInputPorts=12
      settings: ActiveDisplayYMinimum=-1.25  ActiveDisplayYMaximum=1.25
  Triangle Generator{,1..11} (12 alike) : spsTriangleGeneratorLib/Triangle Generator  Freq=5e3  Phase=0  Ts=1e-5
  GateH1 : Outport
  GateH2 : Outport  Port=2
  GateH3 : Outport  Port=3
  GateH4 : Outport  Port=4
  GateH5 : Outport  Port=5
  GateH6 : Outport  Port=6
  wires:
  Mux6/1 -> GateH1/1
  Mux5/1 -> GateH2/1
  Mux4/1 -> GateH3/1
  Mux3/1 -> GateH4/1
  Mux2/1 -> GateH5/1
  Mux1/1 -> GateH6/1
  Relational Operator4/1 -> Mux5/1
  Relational Operator11/1 -> Mux1/2
  Relational Operator10/1 -> Mux2/2
  Relational Operator9/1 -> Mux3/2
  Relational Operator8/1 -> Mux4/2
  Relational Operator7/1 -> Mux5/2
  Relational Operator6/1 -> Mux6/2
  Relational Operator5/1 -> Mux6/1
  Relational Operator3/1 -> Mux4/1
  Relational Operator2/1 -> Mux3/1
  Relational Operator1/1 -> Mux2/1
  Relational Operator/1 -> Mux1/1
  Add12/1 -> Relational Operator11/2, Scope/12
  Add11/1 -> Relational Operator10/2, Scope/11
  Add10/1 -> Relational Operator9/2, Scope/10
  Add9/1 -> Relational Operator8/2, Scope/9
  Add8/1 -> Relational Operator7/2, Scope/8
  Add7/1 -> Relational Operator6/2, Scope/7
  Add6/1 -> Relational Operator5/2, Scope/6
  Add5/1 -> Relational Operator4/2, Scope/5
  Add4/1 -> Relational Operator3/2, Scope/4
  Add3/1 -> Relational Operator2/2, Scope/3
  Add2/1 -> Relational Operator1/2, Scope/2
  Add1/1 -> Relational Operator/2, Scope/1
  Demux/12 -> Add12/1
  Demux/11 -> Add11/1
  Demux/10 -> Add10/1
  Demux/9 -> Add9/1
  Demux/8 -> Add8/1
  Demux/7 -> Add7/1
  Constant9/1 -> Add8/2
  phaa/1 -> Relational Operator/1, Relational Operator1/1, Relational Operator2/1, Relational Operator3/1, Relational Operator4/1, Relational Operator5/1, Relational Operator6/1, Relational Operator7/1, Relational Operator8/1, Relational Operator9/1, Relational Operator10/1, Relational Operator11/1
  Constant11/1 -> Add10/2
  Constant8/1 -> Add7/2
  Constant13/1 -> Add12/2
  Constant10/1 -> Add9/2
  Constant12/1 -> Add11/2
  Triangle Generator11/1 -> Mux/12
  Triangle Generator10/1 -> Mux/11
  Triangle Generator9/1 -> Mux/10
  Triangle Generator8/1 -> Mux/9
  Triangle Generator7/1 -> Mux/8
  Triangle Generator6/1 -> Mux/7
  Add/1 -> Product1/1
  Constant7/1 -> Add6/2
  Demux/6 -> Add6/1
  Constant6/1 -> Add5/2
  Demux/5 -> Add5/1
  Demux/4 -> Add4/1
  Constant5/1 -> Add4/2
  Constant4/1 -> Add3/2
  Demux/3 -> Add3/1
  Demux/2 -> Add2/1
  Constant3/1 -> Add2/2
  Constant2/1 -> Add1/2
  Demux/1 -> Add1/1
  Product1/1 -> Demux/1
  Constant1/1 -> Product1/2
  Constant/1 -> Add/2
  Mux/1 -> Add/1
  Triangle Generator5/1 -> Mux/6
  Triangle Generator4/1 -> Mux/5
  Triangle Generator3/1 -> Mux/4
  Triangle Generator2/1 -> Mux/3
  Triangle Generator1/1 -> Mux/2
  Triangle Generator/1 -> Mux/1

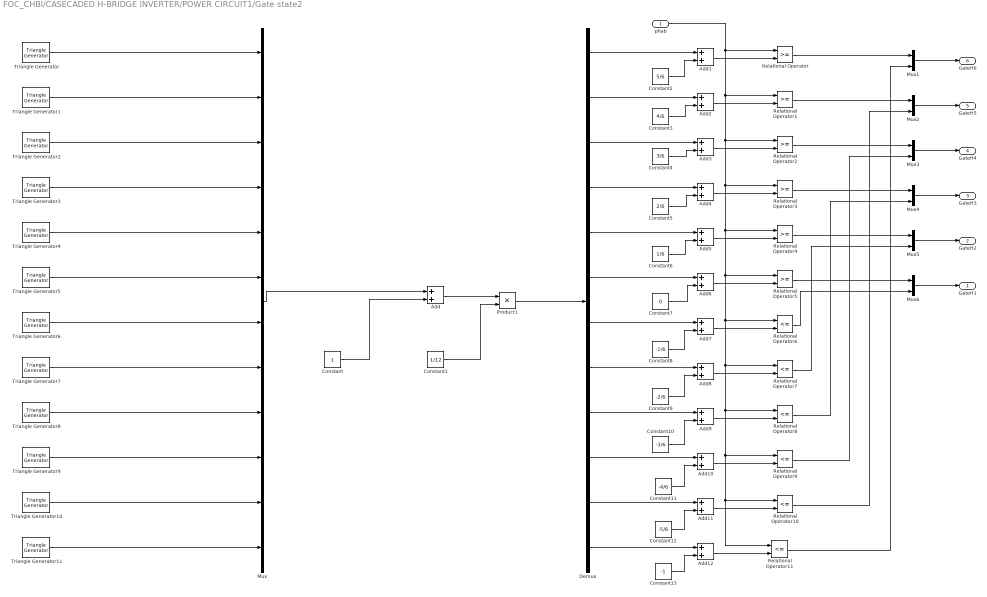
== system FOC_CHBI/CASECADED H-BRIDGE INVERTER/POWER CIRCUIT1/Gate state2  ==
  phab : Inport
  Add{,1..12} (13 alike) : Sum
  Constant : Constant  SampleTime=1e-5
  Constant1 : Constant  Value=1/12  SampleTime=1e-5
  Constant10 : Constant  Value=-3/6  SampleTime=1e-5
  Constant11 : Constant  Value=-4/6  SampleTime=1e-5
  Constant12 : Constant  Value=-5/6  SampleTime=1e-5
  Constant13 : Constant  Value=-1  SampleTime=1e-5
  Constant2 : Constant  Value=5/6  SampleTime=1e-5
  Constant3 : Constant  Value=4/6  SampleTime=1e-5
  Constant4 : Constant  Value=3/6  SampleTime=1e-5
  Constant5 : Constant  Value=2/6  SampleTime=1e-5
  Constant6 : Constant  Value=1/6  SampleTime=1e-5
  Constant7 : Constant  Value=0  SampleTime=1e-5
  Constant8 : Constant  Value=-1/6  SampleTime=1e-5
  Constant9 : Constant  Value=-2/6  SampleTime=1e-5
  Demux : Demux  Outputs=12
  Mux : Mux  Inputs=12
  Mux{1..6} (6 alike) : Mux  Inputs=2
  Product1 : Product
  Relational Operator{,1..5} (6 alike) : RelationalOperator  OutDataTypeStr=boolean  InputSameDT=off
  Relational Operator{6..11} (6 alike) : RelationalOperator  Operator=<=  OutDataTypeStr=boolean  InputSameDT=off
  Triangle Generator{,1..11} (12 alike) : spsTriangleGeneratorLib/Triangle Generator  Freq=5e3  Phase=0  Ts=1e-5
  GateH1 : Outport
  GateH2 : Outport  Port=2
  GateH3 : Outport  Port=3
  GateH4 : Outport  Port=4
  GateH5 : Outport  Port=5
  GateH6 : Outport  Port=6
  wires:
  Triangle Generator7/1 -> Mux/8
  Constant1/1 -> Product1/2
  Relational Operator8/1 -> Mux4/2
  phab/1 -> Relational Operator/1, Relational Operator1/1, Relational Operator2/1, Relational Operator3/1, Relational Operator4/1, Relational Operator5/1, Relational Operator6/1, Relational Operator7/1, Relational Operator8/1, Relational Operator9/1, Relational Operator10/1, Relational Operator11/1
  Add1/1 -> Relational Operator/2
  Demux/1 -> Add1/1
  Product1/1 -> Demux/1
  Triangle Generator8/1 -> Mux/9
  Constant5/1 -> Add4/2
  Constant13/1 -> Add12/2
  Add/1 -> Product1/1
  Add8/1 -> Relational Operator7/2
  Constant7/1 -> Add6/2
  Constant6/1 -> Add5/2
  Relational Operator6/1 -> Mux6/2
  Triangle Generator9/1 -> Mux/10
  Add2/1 -> Relational Operator1/2
  Demux/9 -> Add9/1
  Add4/1 -> Relational Operator3/2
  Constant8/1 -> Add7/2
  Constant2/1 -> Add1/2
  Triangle Generator10/1 -> Mux/11
  Demux/8 -> Add8/1
  Constant11/1 -> Add10/2
  Triangle Generator5/1 -> Mux/6
  Mux4/1 -> GateH3/1
  Constant10/1 -> Add9/2
  Demux/5 -> Add5/1
  Constant9/1 -> Add8/2
  Add6/1 -> Relational Operator5/2
  Add7/1 -> Relational Operator6/2
  Relational Operator9/1 -> Mux3/2
  Demux/6 -> Add6/1
  Add11/1 -> Relational Operator10/2
  Demux/7 -> Add7/1
  Add12/1 -> Relational Operator11/2
  Demux/10 -> Add10/1
  Triangle Generator11/1 -> Mux/12
  Add9/1 -> Relational Operator8/2
  Triangle Generator3/1 -> Mux/4
  Mux2/1 -> GateH5/1
  Triangle Generator2/1 -> Mux/3
  Relational Operator/1 -> Mux1/1
  Relational Operator1/1 -> Mux2/1
  Mux3/1 -> GateH4/1
  Relational Operator2/1 -> Mux3/1
  Demux/11 -> Add11/1
  Demux/12 -> Add12/1
  Constant/1 -> Add/2
  Relational Operator7/1 -> Mux5/2
  Constant3/1 -> Add2/2
  Demux/4 -> Add4/1
  Relational Operator10/1 -> Mux2/2
  Triangle Generator4/1 -> Mux/5
  Mux/1 -> Add/1
  Relational Operator11/1 -> Mux1/2
  Add5/1 -> Relational Operator4/2
  Triangle Generator6/1 -> Mux/7
  Relational Operator4/1 -> Mux5/1
  Add10/1 -> Relational Operator9/2
  Demux/3 -> Add3/1
  Relational Operator5/1 -> Mux6/1
  Relational Operator3/1 -> Mux4/1
  Add3/1 -> Relational Operator2/2
  Mux1/1 -> GateH6/1
  Mux5/1 -> GateH2/1
  Mux6/1 -> GateH1/1
  Constant12/1 -> Add11/2
  Triangle Generator/1 -> Mux/1
  Triangle Generator1/1 -> Mux/2
  Demux/2 -> Add2/1
  Constant4/1 -> Add3/2

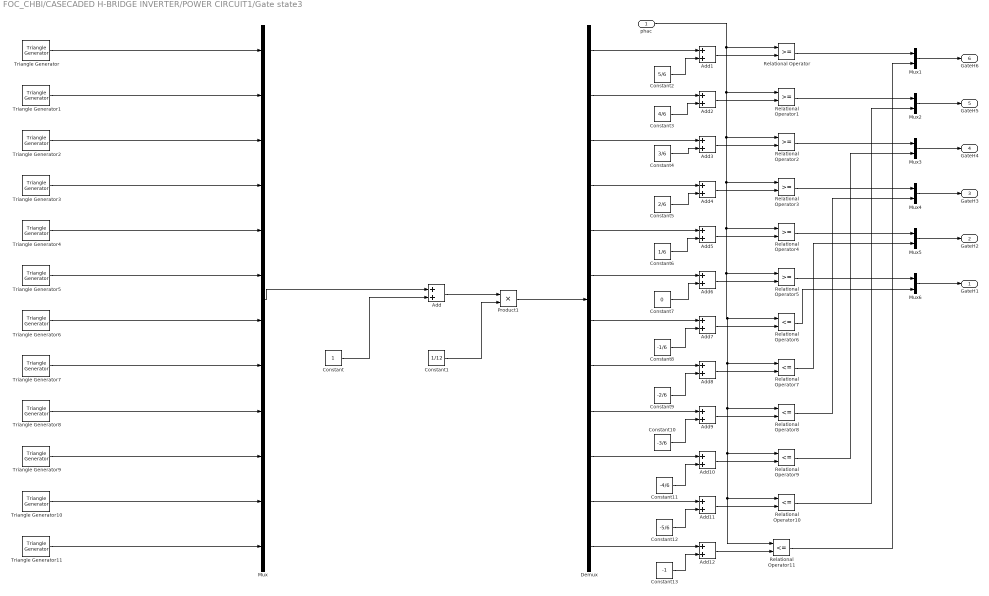
== system FOC_CHBI/CASECADED H-BRIDGE INVERTER/POWER CIRCUIT1/Gate state3 ==
  phac : Inport
  Add{,1..12} (13 alike) : Sum
  Constant : Constant  SampleTime=1e-5
  Constant1 : Constant  Value=1/12  SampleTime=1e-5
  Constant10 : Constant  Value=-3/6  SampleTime=1e-5
  Constant11 : Constant  Value=-4/6  SampleTime=1e-5
  Constant12 : Constant  Value=-5/6  SampleTime=1e-5
  Constant13 : Constant  Value=-1  SampleTime=1e-5
  Constant2 : Constant  Value=5/6  SampleTime=1e-5
  Constant3 : Constant  Value=4/6  SampleTime=1e-5
  Constant4 : Constant  Value=3/6  SampleTime=1e-5
  Constant5 : Constant  Value=2/6  SampleTime=1e-5
  Constant6 : Constant  Value=1/6  SampleTime=1e-5
  Constant7 : Constant  Value=0  SampleTime=1e-5
  Constant8 : Constant  Value=-1/6  SampleTime=1e-5
  Constant9 : Constant  Value=-2/6  SampleTime=1e-5
  Demux : Demux  Outputs=12
  Mux : Mux  Inputs=12
  Mux{1..6} (6 alike) : Mux  Inputs=2
  Product1 : Product
  Relational Operator{,1..5} (6 alike) : RelationalOperator  OutDataTypeStr=boolean  InputSameDT=off
  Relational Operator{6..11} (6 alike) : RelationalOperator  Operator=<=  OutDataTypeStr=boolean  InputSameDT=off
  Triangle Generator{,1..11} (12 alike) : spsTriangleGeneratorLib/Triangle Generator  Freq=5e3  Phase=0  Ts=1e-5
  GateH1 : Outport
  GateH2 : Outport  Port=2
  GateH3 : Outport  Port=3
  GateH4 : Outport  Port=4
  GateH5 : Outport  Port=5
  GateH6 : Outport  Port=6
  wires:
  Triangle Generator7/1 -> Mux/8
  Constant1/1 -> Product1/2
  Relational Operator8/1 -> Mux4/2
  phac/1 -> Relational Operator/1, Relational Operator1/1, Relational Operator2/1, Relational Operator3/1, Relational Operator4/1, Relational Operator5/1, Relational Operator6/1, Relational Operator7/1, Relational Operator8/1, Relational Operator9/1, Relational Operator10/1, Relational Operator11/1
  Add1/1 -> Relational Operator/2
  Demux/1 -> Add1/1
  Product1/1 -> Demux/1
  Triangle Generator8/1 -> Mux/9
  Constant5/1 -> Add4/2
  Constant13/1 -> Add12/2
  Add/1 -> Product1/1
  Add8/1 -> Relational Operator7/2
  Constant7/1 -> Add6/2
  Constant6/1 -> Add5/2
  Relational Operator6/1 -> Mux6/2
  Triangle Generator9/1 -> Mux/10
  Add2/1 -> Relational Operator1/2
  Demux/9 -> Add9/1
  Add4/1 -> Relational Operator3/2
  Constant8/1 -> Add7/2
  Constant2/1 -> Add1/2
  Triangle Generator10/1 -> Mux/11
  Demux/8 -> Add8/1
  Constant11/1 -> Add10/2
  Triangle Generator5/1 -> Mux/6
  Mux4/1 -> GateH3/1
  Constant10/1 -> Add9/2
  Demux/5 -> Add5/1
  Constant9/1 -> Add8/2
  Add6/1 -> Relational Operator5/2
  Add7/1 -> Relational Operator6/2
  Relational Operator9/1 -> Mux3/2
  Demux/6 -> Add6/1
  Add11/1 -> Relational Operator10/2
  Demux/7 -> Add7/1
  Add12/1 -> Relational Operator11/2
  Demux/10 -> Add10/1
  Triangle Generator11/1 -> Mux/12
  Add9/1 -> Relational Operator8/2
  Triangle Generator3/1 -> Mux/4
  Mux2/1 -> GateH5/1
  Triangle Generator2/1 -> Mux/3
  Relational Operator/1 -> Mux1/1
  Relational Operator1/1 -> Mux2/1
  Mux3/1 -> GateH4/1
  Relational Operator2/1 -> Mux3/1
  Demux/11 -> Add11/1
  Demux/12 -> Add12/1
  Constant/1 -> Add/2
  Relational Operator7/1 -> Mux5/2
  Constant3/1 -> Add2/2
  Demux/4 -> Add4/1
  Relational Operator10/1 -> Mux2/2
  Triangle Generator4/1 -> Mux/5
  Mux/1 -> Add/1
  Relational Operator11/1 -> Mux1/2
  Add5/1 -> Relational Operator4/2
  Triangle Generator6/1 -> Mux/7
  Relational Operator4/1 -> Mux5/1
  Add10/1 -> Relational Operator9/2
  Demux/3 -> Add3/1
  Relational Operator5/1 -> Mux6/1
  Relational Operator3/1 -> Mux4/1
  Add3/1 -> Relational Operator2/2
  Mux1/1 -> GateH6/1
  Mux5/1 -> GateH2/1
  Mux6/1 -> GateH1/1
  Constant12/1 -> Add11/2
  Triangle Generator/1 -> Mux/1
  Triangle Generator1/1 -> Mux/2
  Demux/2 -> Add2/1
  Constant4/1 -> Add3/2
